simulink model "Lqg_simulink"  (R2019a)
settings: Solver=VariableStepAuto  StartTime=0.0  StopTime=40  RelTol=1e-3
values from neighbouring files (symbols this model uses):
  A = [0, 0, 1, 0 ... (first row only)    [Base_proyecto.m]    (also in lqr_proyecto.m)
  B = [0 ... (first row only)    [Base_proyecto.m]    (also in lqr_proyecto.m)
  C = [0  1  0  0]    [Base_proyecto.m]    (also in lqr_proyecto.m)
  K = lqr(A,B,Q,R)    [Base_proyecto.m]    (also in lqr_proyecto.m)
  sysKF = ss(A-Kf*C,[B Kf],eye(4),0*[B Kf])    [Base_proyecto.m]
libraries: simulink x1
settings Model: Creator=WALTER  LastModifiedBy=WALTER

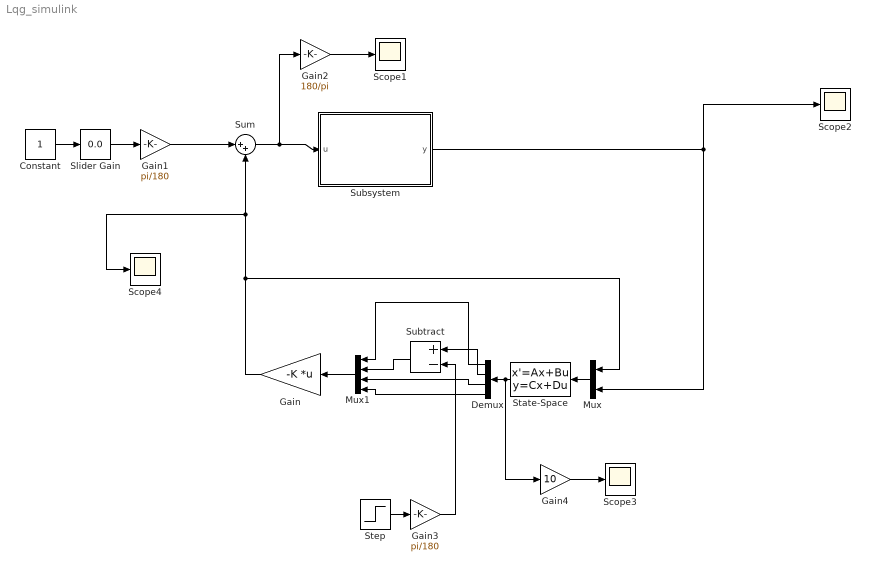
== system Lqg_simulink ==
  Constant : Constant
  Demux : Demux
  Gain : Gain  Gain=-K  Multiplication=Matrix(K*u)
  Gain1 : Gain  Gain=pi/180
  Gain2 : Gain  Gain=180/pi
  Gain3 : Gain  Gain=pi/180
  Gain4 : Gain  Gain=10
  Mux : Mux  Inputs=2
  Mux1 : Mux
  Scope{1..4} (4 alike) : Scope
  Slider Gain : simulink/Math Operations/Slider Gain  gain=0.0  low=-20  high=20
  State-Space : StateSpace  A=sysKF.a  B=sysKF.b  C=sysKF.c  D=sysKF.d  InitialCondition=[0 0 0 0]
  Step : Step  Time=10  SampleTime=5
  Subsystem : Subsystem
  Subtract : Sum  Inputs=+-
  Sum : Sum  Inputs=|++
  wires:
  Gain/1 -> Mux/1, Scope4/1, Sum/2
  Sum/1 -> Gain2/1, Subsystem/1(u)
  Slider Gain/1 -> Gain1/1
  Constant/1 -> Slider Gain/1
  Gain1/1 -> Sum/1
  Gain2/1 -> Scope1/1
  Subsystem/1(y) -> Mux/2, Scope2/1
  Mux/1 -> State-Space/1
  State-Space/1 -> Gain4/1, Demux/1
  Mux1/1 -> Gain/1
  Demux/1 -> Mux1/1
  Step/1 -> Gain3/1
  Demux/3 -> Mux1/3
  Demux/4 -> Mux1/4
  Demux/2 -> Subtract/1
  Subtract/1 -> Mux1/2
  Gain3/1 -> Subtract/2
  Gain4/1 -> Scope3/1

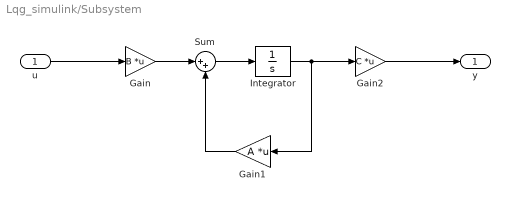
== system Lqg_simulink/Subsystem ==
  u : Inport
  Gain : Gain  Gain=B  Multiplication=Matrix(K*u)
  Gain1 : Gain  Gain=A  Multiplication=Matrix(K*u) (u vector)
  Gain2 : Gain  Gain=C  Multiplication=Matrix(K*u) (u vector)
  Integrator : Integrator
  Sum : Sum  Inputs=|++
  y : Outport
  wires:
  Gain1/1 -> Sum/2
  Gain/1 -> Sum/1
  Integrator/1 -> Gain1/1, Gain2/1
  Gain2/1 -> y/1
  Sum/1 -> Integrator/1
  u/1 -> Gain/1
